simulink model "discreteInner"  (R2020b)
settings: Solver=VariableStepAuto  StartTime=0.0  StopTime=inf  RelTol=2.8421709430404007E-14
values from neighbouring files (symbols this model uses):
  dt_delay = 0.011    [main.m]
  dt_sample = 0.01    [main.m]
  Kd = diag([K1d; K2d; K3d])    [main.m]
  wbi0_B = [0;0;0]    [main.m]
undefined symbols (not defined in the file or in its folder): A_BP, A_PB, J_C_B, K, pd, q0_BI, q_PB, qstar_BI, zd
libraries: dspnetwork x2
settings Model: EnablePacing=on  Creator=bbingham  LastModifiedBy=tjones
settings DataIOCC: SaveOutput=off  SignalLogging=off  DSMLogging=off  ReturnWorkspaceOutputs=off
settings DebuggingCC: ArithmeticOperatorsInVariantConditions=warning
settings SFSimCC: SimUseLocalCustomCode=off  CustomCodeUndefinedFunction=UseInterfaceOnly
settings RTWCC: Description=Simulink Desktop Real-Time  SystemTargetFile=sldrt.tlc  TemplateMakefile=sldrt.tmf  RTWUseLocalCustomCode=off  RTWCompilerOptimization=on
settings CodeAppCC: MaxIdLength=95  StateflowObjectComments=on
settings TargetCC: TargetPreCompLibLocation=C:\Program Files\MATLAB\R2020a\toolbox\sldrt\lib\win64  TargetLangStandard=C99 (ISO)  SupportVariableSizeSignals=on
settings SimscapeCC: SimscapeNormalizeSystem=off

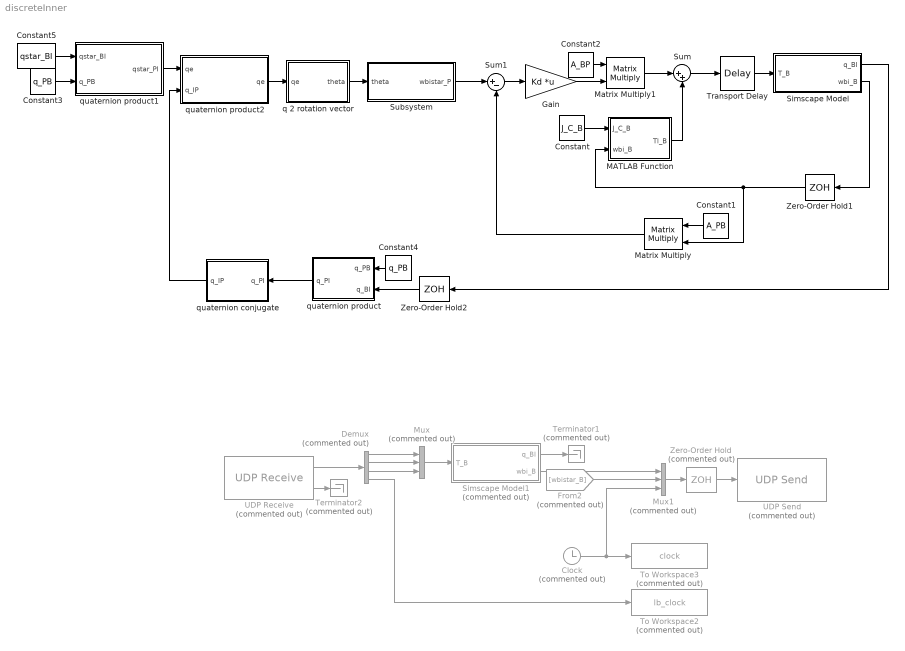
== system discreteInner ==
  Clock : Clock  Commented=on
  Constant : Constant  Value=J_C_B  SampleTime=dt_sample
  Constant1 : Constant  Value=A_PB  SampleTime=dt_sample
  Constant2 : Constant  Value=A_BP  SampleTime=dt_sample
  Constant3 : Constant  Value=q_PB  OutDataTypeStr=Bus: qBus
  Constant4 : Constant  Value=q_PB
  Constant5 : Constant  Value=qstar_BI  OutDataTypeStr=Bus: qBus
  Demux : Demux  Commented=on
  From2 : From  Commented=on  GotoTag=wbistar_B
  Gain : Gain  Gain=Kd  Multiplication=Matrix(K*u) (u vector)
  MATLAB Function : MATLAB Function  TreatAsAtomicUnit=on
  Matrix Multiply : Product  Multiplication=Matrix(*)
  Matrix Multiply1 : Product  Multiplication=Matrix(*)
  Mux : Mux  Commented=on  Inputs=3
  Mux1 : Mux  Commented=on  Inputs=3
  Simscape Model : Subsystem  TreatAsAtomicUnit=on
  Simscape Model1 : Subsystem  Commented=on  TreatAsAtomicUnit=on
  Subsystem : Subsystem
  Sum : Sum  Inputs=|++
  Sum1 : Sum  Inputs=|+-
  Terminator1 : Terminator  Commented=on
  Terminator2 : Terminator  Commented=on
  To Workspace2 : ToWorkspace  Commented=on  VariableName=lb_clock  SaveFormat=Timeseries  SampleTime=-1
  To Workspace3 : ToWorkspace  Commented=on  VariableName=clock  SaveFormat=Timeseries  SampleTime=-1
  Transport Delay : TransportDelay  DelayTime=dt_delay  BufferSize=2048
  UDP Receive : dspnetwork/UDP Receive  Commented=on  localURL='0.0.0.0'  localPort=12346  remoteURL='0.0.0.0'  remotePort=-1  recvBufferSize=8192  dims=4  signalDatatype=double  isComplex=off  isVarSize=off  showBlockingTime=off  blockingTime=0  sampletime=.001  blockPlatform=[]
  UDP Send : dspnetwork/UDP Send  Commented=on  remoteURL='172.31.220.90'  remotePort=12345  localURL='0.0.0.0'  localPortSource=Automatically determine  localPort=-1  sendBufferSize=8192  sampletime=-1  blockPlatform=[]  separateLengthPort=0
  Zero-Order Hold : ZeroOrderHold  Commented=on  SampleTime=dt_sample
  Zero-Order Hold1 : ZeroOrderHold  SampleTime=dt_sample
  Zero-Order Hold2 : ZeroOrderHold  SampleTime=dt_sample
  q 2 rotation vector : MATLAB Function  TreatAsAtomicUnit=on
  quaternion conjugate : MATLAB Function  TreatAsAtomicUnit=on
  quaternion product : MATLAB Function  TreatAsAtomicUnit=on
  quaternion product1 : MATLAB Function  TreatAsAtomicUnit=on
  quaternion product2 : MATLAB Function  TreatAsAtomicUnit=on
  wires:
  Transport Delay/1 -> Simscape Model/1(T_B)
  Simscape Model/1(q_BI) -> Zero-Order Hold2/1
  Sum/1 -> Transport Delay/1
  Zero-Order Hold1/1 -> Matrix Multiply/2, MATLAB Function/2(wbi_B)
  MATLAB Function/1(Tl_B) -> Sum/2
  Constant/1 -> MATLAB Function/1(J_C_B)
  Constant1/1 -> Matrix Multiply/1
  Matrix Multiply/1 -> Sum1/2
  Sum1/1 -> Gain/1
  Constant2/1 -> Matrix Multiply1/1
  Gain/1 -> Matrix Multiply1/2
  Matrix Multiply1/1 -> Sum/1
  Simscape Model/2(wbi_B) -> Zero-Order Hold1/1
  Simscape Model1/1(q_BI) -> Terminator1/1
  UDP Receive/1 -> Demux/1
  Demux/1 -> Mux/1
  Demux/2 -> Mux/2
  Demux/3 -> Mux/3
  Mux/1 -> Simscape Model1/1(T_B)
  UDP Receive/2 -> Terminator2/1
  Simscape Model1/2(wbi_B) -> Mux1/1
  From2/1 -> Mux1/2
  Clock/1 -> To Workspace3/1, Mux1/3
  Demux/4 -> To Workspace2/1
  Mux1/1 -> Zero-Order Hold/1
  Zero-Order Hold/1 -> UDP Send/1
  Zero-Order Hold2/1 -> quaternion product/2(q_BI)
  Constant4/1 -> quaternion product/1(q_PB)
  quaternion product/1(q_PI) -> quaternion conjugate/1(q_PI)
  Constant3/1 -> quaternion product1/2(q_PB)
  quaternion product1/1(qstar_PI) -> quaternion product2/1("qe ")
  quaternion conjugate/1(q_IP) -> quaternion product2/2(q_IP)
  quaternion product2/1(qe) -> q 2 rotation vector/1(qe)
  Subsystem/1(wbistar_P) -> Sum1/1
  q 2 rotation vector/1(theta) -> Subsystem/1(theta)
  Constant5/1 -> quaternion product1/1(qstar_BI)

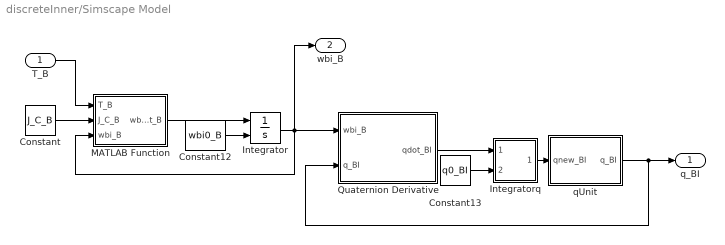
== system discreteInner/Simscape Model ==
  T_B : Inport
  Constant : Constant  Value=J_C_B
  Constant12 : Constant  Value=wbi0_B
  Constant13 : Constant  Value=q0_BI  OutDataTypeStr=Bus: qBus
  Integrator : Integrator  InitialConditionSource=external
  Integratorq : Subsystem
  MATLAB Function : MATLAB Function  TreatAsAtomicUnit=on
  Quaternion Derivative : MATLAB Function  TreatAsAtomicUnit=on
  qUnit : MATLAB Function  TreatAsAtomicUnit=on
  q_BI : Outport  OutDataTypeStr=Bus: qBus  VectorParamsAs1DForOutWhenUnconnected=off
  wbi_B : Outport  Port=2  VectorParamsAs1DForOutWhenUnconnected=off
  wires:
  qUnit/1(q_BI) -> q_BI/1, Quaternion Derivative/2(q_BI)
  Integratorq/1(qnew_BI) -> qUnit/1(qnew_BI)
  Quaternion Derivative/1(qdot_BI) -> Integratorq/1(qdot_BI)
  Constant13/1 -> Integratorq/2(q0_BI)
  MATLAB Function/1(wbidot_B) -> Integrator/1
  Constant12/1 -> Integrator/2
  Constant/1 -> MATLAB Function/2(J_C_B)
  Integrator/1 -> wbi_B/1, MATLAB Function/3(wbi_B), Quaternion Derivative/1(wbi_B)
  T_B/1 -> MATLAB Function/1(T_B)

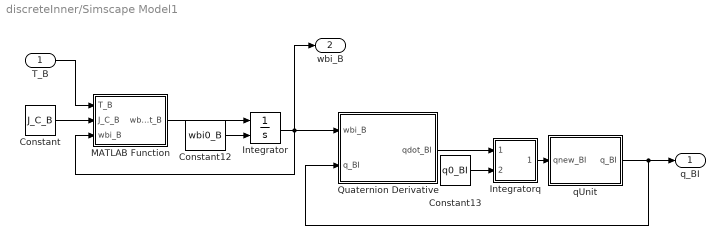
== system discreteInner/Simscape Model1 ==
  T_B : Inport
  Constant : Constant  Value=J_C_B
  Constant12 : Constant  Value=wbi0_B
  Constant13 : Constant  Value=q0_BI  OutDataTypeStr=Bus: qBus
  Integrator : Integrator  InitialConditionSource=external
  Integratorq : Subsystem
  MATLAB Function : MATLAB Function  TreatAsAtomicUnit=on
  Quaternion Derivative : MATLAB Function  TreatAsAtomicUnit=on
  qUnit : MATLAB Function  TreatAsAtomicUnit=on
  q_BI : Outport  OutDataTypeStr=Bus: qBus  VectorParamsAs1DForOutWhenUnconnected=off
  wbi_B : Outport  Port=2  VectorParamsAs1DForOutWhenUnconnected=off
  wires:
  T_B/1 -> MATLAB Function/1(T_B)
  Integrator/1 -> Quaternion Derivative/1(wbi_B), MATLAB Function/3(wbi_B), wbi_B/1
  Constant/1 -> MATLAB Function/2(J_C_B)
  Constant12/1 -> Integrator/2
  MATLAB Function/1(wbidot_B) -> Integrator/1
  Constant13/1 -> Integratorq/2(q0_BI)
  Quaternion Derivative/1(qdot_BI) -> Integratorq/1(qdot_BI)
  Integratorq/1(qnew_BI) -> qUnit/1(qnew_BI)
  qUnit/1(q_BI) -> Quaternion Derivative/2(q_BI), q_BI/1

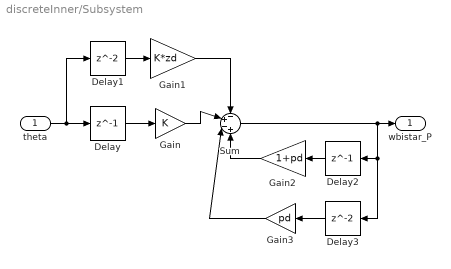
== system discreteInner/Subsystem ==
  theta : Inport
  Delay : Delay  DelayLength=1
  Delay1 : Delay
  Delay2 : Delay  DelayLength=1
  Delay3 : Delay
  Gain : Gain  Gain=K
  Gain1 : Gain  Gain=K*zd
  Gain2 : Gain  Gain=1+pd
  Gain3 : Gain  Gain=pd
  Sum : Sum  Inputs=-+-+
  wbistar_P : Outport
  wires:
  Sum/1 -> Delay3/1, Delay2/1, wbistar_P/1
  theta/1 -> Delay1/1, Delay/1
  Gain/1 -> Sum/2
  Delay/1 -> Gain/1
  Delay1/1 -> Gain1/1
  Gain1/1 -> Sum/1
  Delay2/1 -> Gain2/1
  Gain2/1 -> Sum/4
  Delay3/1 -> Gain3/1
  Gain3/1 -> Sum/3

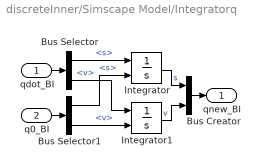
== system discreteInner/Simscape Model/Integratorq ==
  qdot_BI : Inport  OutDataTypeStr=Bus: qBus
  q0_BI : Inport  Port=2  OutDataTypeStr=Bus: qBus
  Bus Creator : BusCreator  Inputs=2  OutDataTypeStr=Bus: qBus
      settings: InheritFromInputs=off
  Bus Selector : BusSelector  OutputSignals=s,v
  Bus Selector1 : BusSelector  OutputSignals=s,v
  Integrator : Integrator  InitialConditionSource=external
  Integrator1 : Integrator  InitialConditionSource=external
  qnew_BI : Outport  OutDataTypeStr=Bus: qBus  VectorParamsAs1DForOutWhenUnconnected=off
  wires:
  qdot_BI/1 -> Bus Selector/1
  q0_BI/1 -> Bus Selector1/1
  Bus Selector/1 -> Integrator/1  "<s>"
  Bus Selector1/1 -> Integrator/2  "<s>"
  Bus Selector/2 -> Integrator1/1  "<v>"
  Bus Selector1/2 -> Integrator1/2  "<v>"
  Integrator/1 -> Bus Creator/1  "s"
  Integrator1/1 -> Bus Creator/2  "v"
  Bus Creator/1 -> qnew_BI/1

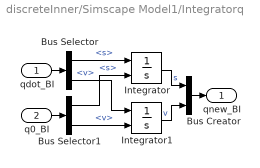
== system discreteInner/Simscape Model1/Integratorq ==
  qdot_BI : Inport  OutDataTypeStr=Bus: qBus
  q0_BI : Inport  Port=2  OutDataTypeStr=Bus: qBus
  Bus Creator : BusCreator  Inputs=2  OutDataTypeStr=Bus: qBus
      settings: InheritFromInputs=off
  Bus Selector : BusSelector  OutputSignals=s,v
  Bus Selector1 : BusSelector  OutputSignals=s,v
  Integrator : Integrator  InitialConditionSource=external
  Integrator1 : Integrator  InitialConditionSource=external
  qnew_BI : Outport  OutDataTypeStr=Bus: qBus  VectorParamsAs1DForOutWhenUnconnected=off
  wires:
  Bus Creator/1 -> qnew_BI/1
  Integrator1/1 -> Bus Creator/2  "v"
  Integrator/1 -> Bus Creator/1  "s"
  Bus Selector1/2 -> Integrator1/2  "<v>"
  Bus Selector/2 -> Integrator1/1  "<v>"
  Bus Selector1/1 -> Integrator/2  "<s>"
  Bus Selector/1 -> Integrator/1  "<s>"
  q0_BI/1 -> Bus Selector1/1
  qdot_BI/1 -> Bus Selector/1

== matlab function discreteInner/MATLAB Function ==
  data: J_C_B input; Tl_B output; wbi_B input
function Tl_B = fcn(J_C_B, wbi_B)

Tl_B = cross(wbi_B, J_C_B*wbi_B);

== matlab function discreteInner/Simscape Model/Quaternion Derivative ==
  data: wbi_B input; q_BI input Bus: qBus; qdot_BI output Bus: qBus
function qdot_BI = fcn(wbi_B, q_BI)

w.s = 0;
w.v = wbi_B;

qdot = qX(w, q_BI);

qdot_BI.s = 1/2*qdot.s;
qdot_BI.v = 1/2*qdot.v;

== matlab function discreteInner/Simscape Model1/MATLAB Function ==
  data: T_B input; wbidot_B output; J_C_B input; wbi_B input
function wbidot_B = fcn(T_B, J_C_B, wbi_B)

wbidot_B = J_C_B\(T_B - cross(wbi_B, J_C_B*wbi_B));

== matlab function discreteInner/Simscape Model1/Quaternion Derivative ==
  data: wbi_B input; q_BI input Bus: qBus; qdot_BI output Bus: qBus
function qdot_BI = fcn(wbi_B, q_BI)

w.s = 0;
w.v = wbi_B;

qdot = qX(w, q_BI);

qdot_BI.s = 1/2*qdot.s;
qdot_BI.v = 1/2*qdot.v;

== matlab function discreteInner/Simscape Model1/qUnit ==
  data: qnew_BI input Bus: qBus; q_BI output Bus: qBus
function q_BI = fcn(qnew_BI)

q_BI = qUnit(qnew_BI);

== matlab function discreteInner/quaternion product ==
  data: q_PB input; q_PI output; q_BI input
function q_PI = fcn(q_PB, q_BI)

q_PI = qX(q_PB, q_BI);

== matlab function discreteInner/quaternion conjugate ==
  data: q_PI input; q_IP output
function q_IP = fcn(q_PI)

q_IP = qT(q_PI);

== matlab function discreteInner/quaternion product1 ==
  data: qstar_BI input; q_PB input; qstar_PI output
function qstar_PI = fcn(qstar_BI, q_PB)

qstar_PI = qX(qstar_BI, q_PB);

== matlab function discreteInner/quaternion product2 ==
  data: qe input; qe output; q_IP input
function qe = fcn(qe, q_IP)

qe = qX(qe, q_IP);

== matlab function discreteInner/q 2 rotation vector ==
  data: qe input; theta output
function theta = fcn(qe)

[e, th] = q2e(qe);

theta = th*e;

== matlab function discreteInner/Simscape Model/MATLAB Function ==
  data: T_B input; wbidot_B output; J_C_B input; wbi_B input
function wbidot_B = fcn(T_B, J_C_B, wbi_B)

wbidot_B = J_C_B\(T_B - cross(wbi_B, J_C_B*wbi_B));

== matlab function discreteInner/Simscape Model/qUnit ==
  data: qnew_BI input Bus: qBus; q_BI output Bus: qBus
function q_BI = fcn(qnew_BI)

q_BI = qUnit(qnew_BI);
